simulink model "THIS_WORKS_YAY_previous_version"  (R2019b)
settings: Solver=ode8  StartTime=0.0  StopTime=tfinal  FixedStep=0.1  RelTol=1e-3
values from neighbouring files (symbols this model uses):
  ax_zero = ReqVar.Max_Acceleration    [All_inputs.m]
  Cd = ReqVar.Coefficient_Of_Drag    [All_inputs.m]    (also in Run_This1.m; Velocity_Profile.m; trial6.m)
  Frontal_Area = ReqVar.Frontal_Area    [All_inputs.m]    (also in Run_This1.m; Velocity_Profile.m)
  g = 9.80665    [Run_This.m]    (also in Run_This1.m; Velocity_Profile.m; trial6.m)
  Gear_Ratio = ReqVar.Gear_Ratio    [All_inputs.m]    (also in Run_This1.m; Velocity_Profile.m; trial6.m)
  N = length(rho_v_filter1)    [Attempt.m]    (also in B1654run24.mat = [480.23 479.95 479.61 479.47 479.27 479.41 479.68 480.02 480; Comp_Input.m; DataInput.m = FILE(:,3); ImportRawData.m = lat_test.data(:,3))
  Roll_Res = ReqVar.Roll_Res    [All_inputs.m]    (also in Run_This1.m; Velocity_Profile.m; trial6.m)
  T0 = ReqVar.T0    [All_inputs.m]    (also in Run_This1.m; Velocity_Profile.m; trial6.m)
  Tire_Radius = ReqVar.Tire_radius    [All_inputs.m]    (also in Run_This1.m; Velocity_Profile.m)
  v_max = v_max/3.6    [All_inputs.m]    (also in Run_This1.m; Velocity_Profile.m)
  v_new = (1:N)    [Run_This1.m]    (also in Velocity_Profile.m; trial6.m)
  W = m    [All_inputs.m]    (also in Velocity_Profile.m)
libraries: simulink x1, autolibshared x1
settings Model: Creator=adith  LastModifiedBy=Admin
settings SFSimCC: CustomCodeUndefinedFunction=UseInterfaceOnly

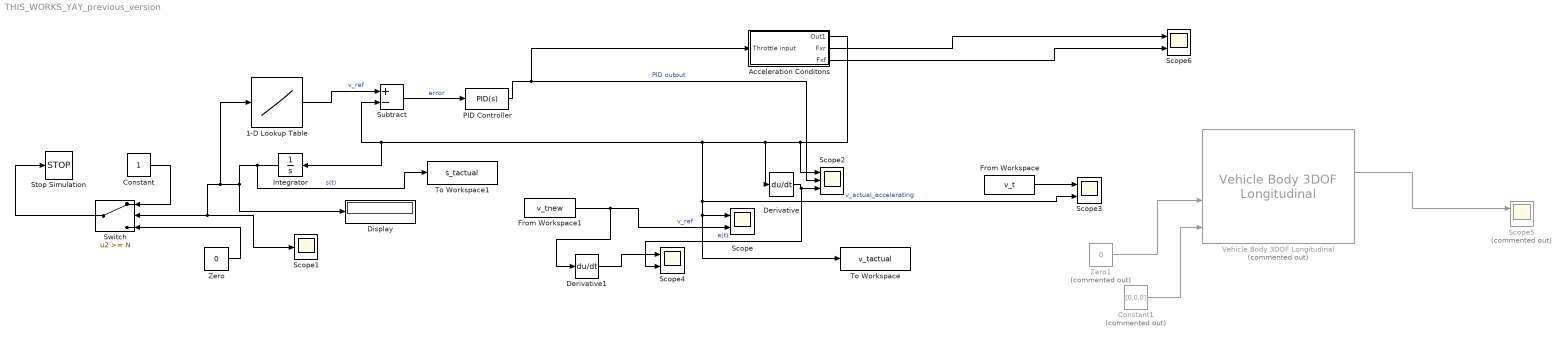
== system THIS_WORKS_YAY_previous_version ==
  1-D Lookup Table : Lookup_n-D  NumberOfTableDimensions=1  LookupTableObject=v_new  BreakpointsForDimension1=[1:N]  Table=v_new  InternalRulePriority=Speed  RndMeth=Simplest  InputSameDT=on
  Acceleration Conditons : Subsystem
  Constant : Constant
  Constant1 : Constant  Commented=on  Value=[0,0,0]
  Derivative : Derivative
  Derivative1 : Derivative
  Display : Display
  From Workspace : FromWorkspace  VariableName=v_t  SampleTime=0
  From Workspace1 : FromWorkspace  VariableName=v_tnew  SampleTime=0
  Integrator : Integrator
  PID Controller : simulink/Continuous/PID Controller  Controller=PID  Form=Parallel  TimeDomain=Continuous-time  SampleTime=-1  IntegratorMethod=Forward Euler  FilterMethod=Forward Euler  ControllerParametersSource=internal  P=3  I=0  D=0  UseFilter=on  N=0.174097503421511  TunerSelectOption=Transfer Function Based (PID Tuner App)  InitialConditionSource=internal  InitialConditionForIntegrator=0  InitialConditionForFilter=0  DifferentiatorICPrevScaledInput=0  ExternalReset=none  TrackingMode=off  Kt=1  LimitOutput=on  UpperSaturationLimit=1  LowerSaturationLimit=-1  LinearizeAsGain=on  AntiWindupMode=none  Kb=1  POutMin=[]  POutMax=[]  IOutMin=[]  IOutMax=[]  DOutMin=[]  DOutMax=[]  NOutMin=[]  NOutMax=[]  SumOutMin=[]  SumOutMax=[]  SaturationOutMin=[]  SaturationOutMax=[]  PParamMin=[]  PParamMax=[]  IParamMin=[]  IParamMax=[]  DParamMin=[]  DParamMax=[]  NParamMin=[]  NParamMax=[]  KbParamMin=[]  KbParamMax=[]  KtParamMin=[]  KtParamMax=[]  KbOutMin=[]  KbOutMax=[]  KtOutMin=[]  KtOutMax=[]  IntegratorOutMin=[]  IntegratorOutMax=[]  FilterOutMin=[]  FilterOutMax=[]  SumI1OutMin=[]  SumI1OutMax=[]  SumI2OutMin=[]  SumI2OutMax=[]  SumI3OutMin=[]  SumI3OutMax=[]  SumI4OutMin=[]  SumI4OutMax=[]  SumDOutMin=[]  SumDOutMax=[]  DifferentiatorOutMin=[]  DifferentiatorOutMax=[]  FilterDiffOutCoefMin=[]  FilterDiffOutCoefMax=[]  ReciprocalOutMin=[]  ReciprocalOutMax=[]  SumDenOutMin=[]  SumDenOutMax=[]  SumNumOutMin=[]  SumNumOutMax=[]  DivideOutMin=[]  DivideOutMax=[]  IntegratorContinuousStateAttributes=''  IntegratorStateMustResolveToSignalObject=off  IntegratorRTWStateStorageClass=Auto  FilterContinuousStateAttributes=''  FilterStateMustResolveToSignalObject=off  FilterRTWStateStorageClass=Auto  ParallelPVariant=InternalParameters  IdealPVariant=Disabled  IVariant=InternalParameters  DVariant=InternalParameters  IntegratorVariant=Continuous  SatVariant=Enabled  AWVariant=Passthrough  PCopyVariant=Disabled  TRVariant=Disabled  FdbkBlocksVariant=Forward  IdealPFdbkVariant=Disabled  SatFdbkVariant=Disabled  DerivativeFilterVariant=ContFilter  NVariant=InternalParameters  NCopyVariant=Disabled  FilterICVariant=InternalICsFilter  IntegratorICVariant=InternalICs  ExternalResetVariant=Disabled  TRSumVariant=Passthrough  SumFdbkVariant=Disabled  SumVariant=Sum_PID
  Scope{,3..4,6} (4 alike) : Scope  NumInputPorts=2
  Scope1 : Scope
  Scope2 : Scope  NumInputPorts=3
  Scope5 : Scope  Commented=on  NumInputPorts=2
  Stop Simulation : Stop
  Subtract : Sum  Inputs=+-
  Switch : Switch  Threshold=N
  To Workspace : ToWorkspace  VariableName=v_tactual  SampleTime=-1
      settings: Save2DSignal=2-D array (concatenate along first dimension)
  To Workspace1 : ToWorkspace  VariableName=s_tactual  SampleTime=-1
      settings: Save2DSignal=2-D array (concatenate along first dimension)
  Vehicle Body 3DOF Longitudinal : autolibshared/Vehicle Body 3DOF Longitudinal  Commented=on  VariantControl=SL  groundType=Grade angle  aMode=1  extFMode=off  extMMode=off  extTamb=off  NF=1  NR=1  m=320  a=1.4  b=1.8  h=.35  Cd=.3  Af=Frontal_Area  x_o=0  xdot_o=v_max  Cl=Coefficient_Of_Lift  z_o=-.35  zdot_o=0  Iyy=3500  Cpm=.1  theta_o=0  q_o=0  FskF=[-50, -1, 0, 2, 3, 52].*1.5e4  dzsF=[-5e-3, -1e-4, 0, .2, .2001, .2051]  FsbF=[-10000 -100 -10 0 10 100 10000]  dzdotsF=[-10 -1 -.1 0 .1 1 10]  FskR=[-50, -1, 0, 2, 3, 52].*1e4  dzsR=[-5e-3, -1e-4, 0, .2, .2001, .2051]  FsbR=[-10000 -100 -10 0 10 100 10000]  dzdotsR=[-10 -1 -.1 0 .1 1 10]  Pabs=101325  T=273  g=9.81  blkID=0
      settings: SourceProductName=Powertrain Blockset  SourceProductBaseCode=PW
  Zero : Constant  Value=0  OutDataTypeStr=Inherit: Inherit via back propagation
  Zero1 : Constant  Commented=on  Value=0  OutDataTypeStr=Inherit: Inherit via back propagation
  wires:
  Acceleration Conditons/1(Out1) -> Derivative/1, Scope3/2, To Workspace/1, Scope/1, Integrator/1, Subtract/2, Scope2/1  "v_actual_accelerating"
  PID Controller/1 -> Scope2/2, Acceleration Conditons/1(Throttle input)  "PID output"
  Subtract/1 -> PID Controller/1  "error"
  Integrator/1 -> To Workspace1/1, Display/1, 1-D Lookup Table/1, Scope1/1, Switch/2  "s(t)"
  Switch/1 -> Stop Simulation/1
  Constant/1 -> Switch/1
  Zero/1 -> Switch/3
  From Workspace1/1 -> Derivative1/1, Scope/2  "v_ref"
  1-D Lookup Table/1 -> Subtract/1  "v_ref"
  Derivative/1 -> Scope4/2, Scope2/3  "a(t)"
  From Workspace/1 -> Scope3/1
  Derivative1/1 -> Scope4/1
  Acceleration Conditons/2(Fxr) -> Scope6/1
  Zero1/1 -> Vehicle Body 3DOF Longitudinal/3
  Constant1/1 -> Vehicle Body 3DOF Longitudinal/4
  Vehicle Body 3DOF Longitudinal/2 -> Scope5/1
  Acceleration Conditons/3(Fxf) -> Scope6/2

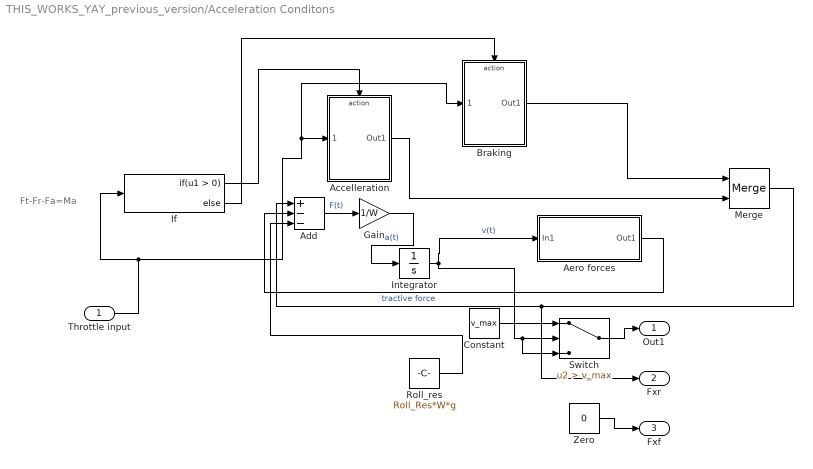
== system THIS_WORKS_YAY_previous_version/Acceleration Conditons ==
  note: Ft-Fr-Fa=Ma
  Throttle input : Inport
  Accelleration : Subsystem  TreatAsAtomicUnit=on
  Add : Sum  Inputs=+--
  Aero forces : Subsystem
  Braking : Subsystem  TreatAsAtomicUnit=on
  Constant : Constant  Value=v_max
  Gain : Gain  Gain=1/W
  If : If
  Integrator : Integrator  InitialCondition=v_max
  Merge : Merge
  Roll_res : Constant  Value=Roll_Res*W*g
  Switch : Switch  Criteria=u2 > Threshold  Threshold=v_max
  Zero : Constant  Value=0  OutDataTypeStr=Inherit: Inherit via back propagation
  Out1 : Outport
  Fxr : Outport  Port=2
  Fxf : Outport  Port=3
  wires:
  Throttle input/1 -> If/1, Braking/1(Throttle input), Accelleration/1(Throttle input)
  Integrator/1 -> Switch/3, Switch/2, Aero forces/1(In1)  "v(t)"
  Roll_res/1 -> Add/3
  Aero forces/1(Out1) -> Add/2
  Add/1 -> Gain/1  "F(t)"
  Gain/1 -> Integrator/1  "a(t)"
  If/1 -> Accelleration/Action
  If/2 -> Braking/Action
  Braking/1(Out1) -> Merge/1
  Accelleration/1(Out1) -> Merge/2
  Merge/1 -> Fxr/1, Add/1  "tractive force"
  Constant/1 -> Switch/1
  Switch/1 -> Out1/1
  Zero/1 -> Fxf/1

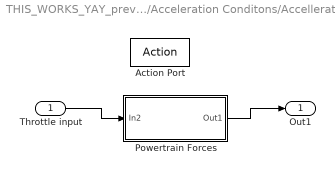
== system THIS_WORKS_YAY_previous_version/Acceleration Conditons/Accelleration ==
  Throttle input : Inport
  Action Port : ActionPort  ActionPortLabel=if(u1 > 0)
  Powertrain Forces : Subsystem
  Out1 : Outport
  wires:
  Throttle input/1 -> Powertrain Forces/1(In2)
  Powertrain Forces/1(Out1) -> Out1/1

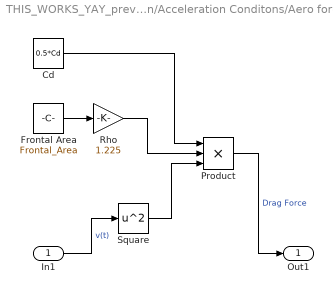
== system THIS_WORKS_YAY_previous_version/Acceleration Conditons/Aero forces ==
  In1 : Inport
  Cd : Constant  Value=0.5*Cd
  Frontal Area : Constant  Value=Frontal_Area
  Product : Product  Inputs=3
  Rho : Gain  Gain=1.225
  Square : Math  Operator=square  SaturateOnIntegerOverflow=on
  Out1 : Outport
  wires:
  In1/1 -> Square/1  "v(t)"
  Frontal Area/1 -> Rho/1
  Cd/1 -> Product/1
  Rho/1 -> Product/2
  Square/1 -> Product/3
  Product/1 -> Out1/1  "Drag Force"

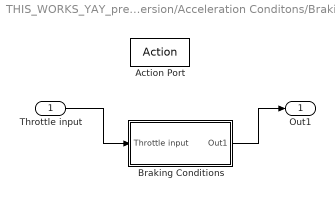
== system THIS_WORKS_YAY_previous_version/Acceleration Conditons/Braking ==
  Throttle input : Inport
  Action Port : ActionPort  ActionPortLabel=else
  Braking Conditions : Subsystem
  Out1 : Outport
  wires:
  Throttle input/1 -> Braking Conditions/1(Throttle input)
  Braking Conditions/1(Out1) -> Out1/1

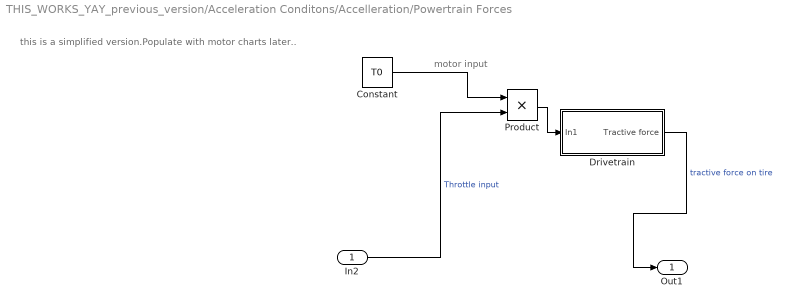
== system THIS_WORKS_YAY_previous_version/Acceleration Conditons/Accelleration/Powertrain Forces ==
  note: motor input
  note: this is a simplified version.Populate with motor charts later..
  In2 : Inport
  Constant : Constant  Value=T0
  Drivetrain : Subsystem
  Product : Product
  Out1 : Outport
  wires:
  In2/1 -> Product/2  "Throttle input"
  Constant/1 -> Product/1
  Product/1 -> Drivetrain/1(In1)
  Drivetrain/1(Tractive force) -> Out1/1  "tractive force on tire"

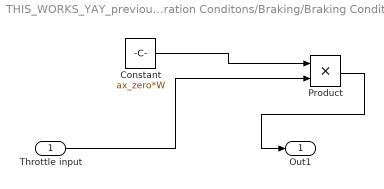
== system THIS_WORKS_YAY_previous_version/Acceleration Conditons/Braking/Braking Conditions ==
  Throttle input : Inport
  Constant : Constant  Value=ax_zero*W
  Product : Product
  Out1 : Outport
  wires:
  Throttle input/1 -> Product/2
  Constant/1 -> Product/1
  Product/1 -> Out1/1

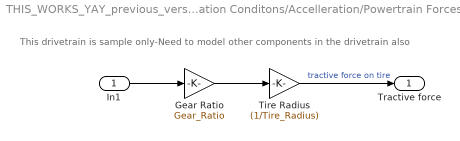
== system THIS_WORKS_YAY_previous_version/Acceleration Conditons/Accelleration/Powertrain Forces/Drivetrain ==
  note: This drivetrain is sample only-Need to model other components in the drivetrain also
  In1 : Inport
  Gear Ratio : Gain  Gain=Gear_Ratio
  Tire Radius : Gain  Gain=(1/Tire_Radius)
  Tractive force : Outport
  wires:
  In1/1 -> Gear Ratio/1
  Gear Ratio/1 -> Tire Radius/1
  Tire Radius/1 -> Tractive force/1  "tractive force on tire"
